simulink model "modelo_n_linear"  (R2023a)
settings: Solver=ode45  StartTime=0.0  StopTime=10.0  MaxStep=0.01  RelTol=1e-3
model workspace: external: MATLAB File C:\Users\pinki\OneDrive\aviãozinho\monociclo\numvars.m (data not in the file)
settings Model: Creator=pinki  LastModifiedBy=pinki
settings DataIOCC: InspectSignalLogs=on

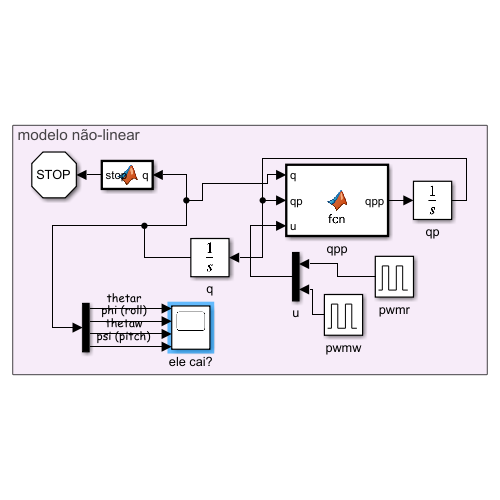
[thumbnail: Simulink's stored preview of the top-level diagram]
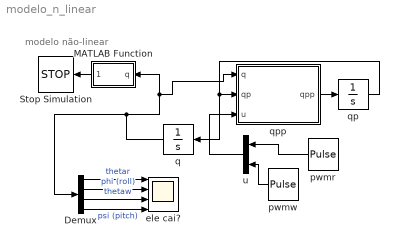
== system modelo_n_linear ==
  note: modelo não-linear
  Demux : Demux
  MATLAB Function : MATLAB Function  TreatAsAtomicUnit=on
  Stop Simulation : Stop
  ele cai? : Scope  NumInputPorts=4
  pwmr : DiscretePulseGenerator  PulseType=Time based  Amplitude=12  Period=1  PulseWidth=5
  pwmw : DiscretePulseGenerator  PulseType=Time based  Amplitude=12  Period=1  PulseWidth=5
  q : Integrator  InitialCondition=[0.05;0.1;0.004;0.07]  ContinuousStateAttributes='q'
  qp : Integrator  InitialCondition=[0;0;0;0]  ContinuousStateAttributes='qp'
  qpp : MATLAB Function  Description=nonlinear model  TreatAsAtomicUnit=on
  u : Mux  Inputs=2
  wires:
  qpp/1(qpp) -> qp/1
  pwmr/1 -> u/1
  u/1 -> qpp/3(u)
  pwmw/1 -> u/2
  Demux/1 -> ele cai?/1  "thetar"
  Demux/2 -> ele cai?/2  "phi (roll)"
  Demux/3 -> ele cai?/3  "thetaw"
  Demux/4 -> ele cai?/4  "psi (pitch)"
  q/1 -> Demux/1, qpp/1(q), MATLAB Function/1(q)
  qp/1 -> q/1, qpp/2(qp)
  MATLAB Function/1(stop) -> Stop Simulation/1

== matlab function modelo_n_linear/MATLAB Function ==
  data: q input; stop output
function stop = fcn(q)

Roll = q(2);
Pitch = q(4);

%% assumindo deslocamento m'aximo de 30 graus ou 0,5 rad...
limite = 0.5;

stop = abs(Pitch)>limite || abs(Roll)>limite;

== matlab function modelo_n_linear/qpp ==
  data: q input; qp input; qpp output; u input
function qpp= fcn(q,qp,u)
%% setup
mono = monociclo;

thetar = q(1);
thetarp = qp(1);

phi = q(2);
phip = qp(2);

thetaw = q(3);
thetawp = qp(3);

psi = q(4);
psip = qp(4);

%% matriz m
m11 = mono.jr;
m12 = m11;
m21 = m11;
m22 = (mono.jbw+mono.jr+(mono.mb+mono.mr+mono.mw)*mono.rw^2 ...
+2*(mono.l*(mono.mb*mono.rw+mono.mr*mono.rw)+mono.mr*mono.rw*mono.d)*cos(psi)...
+(mono.l^2*(mono.mb+mono.mr)+mono.mr*mono.d^2+2*mono.l*mono.mr*mono.d)*cos(psi)^2);
m33 = mono.jw+(mono.mb+mono.mr+mono.mw)*mono.rw^2;
m34 = mono.rw*cos(psi)*(mono.mr*mono.d+mono.l*mono.mb+mono.l*mono.mr);
m43 = m34;
m44 = mono.jbr+mono.mb*mono.l^2+mono.mr*mono.l^2+mono.mr*mono.d^2 ...
    +2*mono.l*mono.mr*mono.d;

M = zeros(4,4);
    M(1,1) = m11;
    M(1,2) = m12;
    M(2,1) = m21;
    M(2,2) = m22;
    M(3,3) = m33;
    M(3,4) = m34;
    M(4,3) = m43;
    M(4,4) = m44;

%% matriz v
v1 = (mono.ker*mono.ktr*mono.nr*(mono.nr*thetarp))/mono.rer ...
     - mono.bvr*thetar;
v2 = -(mono.ker*mono.ktr*mono.nr*(mono.nr*thetarp))/mono.rer ...
     - 2*(mono.l*mono.mb+mono.mr*mono.d)*mono.rw*phip*psip*sin(psi) ...
     - (mono.mr*mono.l^2+mono.mb*mono.l^2+mono.mr*mono.d^2+2*mono.l*mono.mr*mono.d)*phip*psip*sin(2*psi) ...
     - mono.bvr*thetar;
v3 = (mono.ker*mono.ktw*mono.nw*(mono.nw*thetawp-psip))/mono.rew ...
    + (mono.l*mono.mb+mono.d*mono.mr+mono.l*mono.mr)*mono.rw*psip^2*sin(psi) ...
    + mono.bvw*thetaw;
v4 = -(mono.ker*mono.ktw*mono.nw*(mono.nw*thetawp-psip))/mono.rew ...
    + (mono.l*mono.mb+mono.d*mono.mr+mono.l*mono.mr)*mono.rw*phip^2*sin(psi) ...
    + (sin(2*psi)*phip^2*((mono.mb*mono.l^2)+(mono.mr*mono.l^2) ...
    + (mono.mr*mono.d^2))/2+mono.l*mono.mr*mono.d)+mono.bvw*thetaw;

V = zeros(4,1);
    V(1) = v1;
    V(2) = v2;
    V(3) = v3;
    V(4) = v4;

%% matriz g
g2 = -mono.g*sin(phi)*((mono.mb+mono.mr+mono.mw)*mono.rw+(mono.l*mono.mb ...
    + mono.l*mono.mr + mono.mr*mono.d)*cos(psi));
g4 = -mono.g*cos(phi)*sin(psi)*(mono.mr*mono.d+mono.l*mono.mb+mono.l*mono.mr);

G = zeros(4,1);
    G(2) = g2;
    G(4) = g4;

%% matriz p
p11 = (12*mono.ktr*mono.nr)/mono.rr;
p12 = -p11;
p23 = (12*mono.ktw*mono.nw)/mono.rw;
p24 = -p23;

P = zeros(4,2);
    P(1,1) = p11;
    P(2,1) = p12;
    P(3,2) = p23;
    P(4,2) = p24;

%% qpp
qpp = M\(-V-G+P*u);
